simulink model "carSimulation_model"  (R2025b)
settings: Solver=VariableStepAuto  StartTime=0.0  StopTime=1000  RelTol=1e-3
settings Model: Creator=Eddy  LastModifiedBy=Eddy

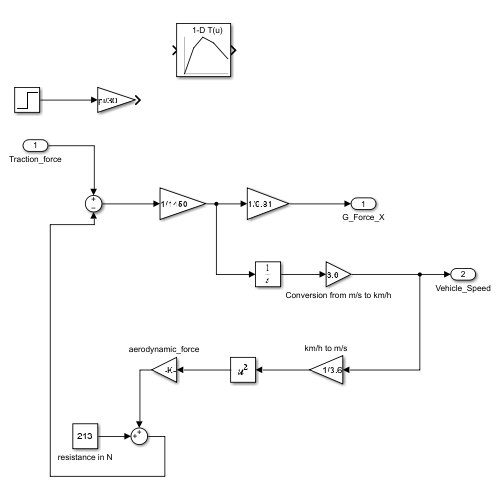
[thumbnail: Simulink's stored preview of the top-level diagram]
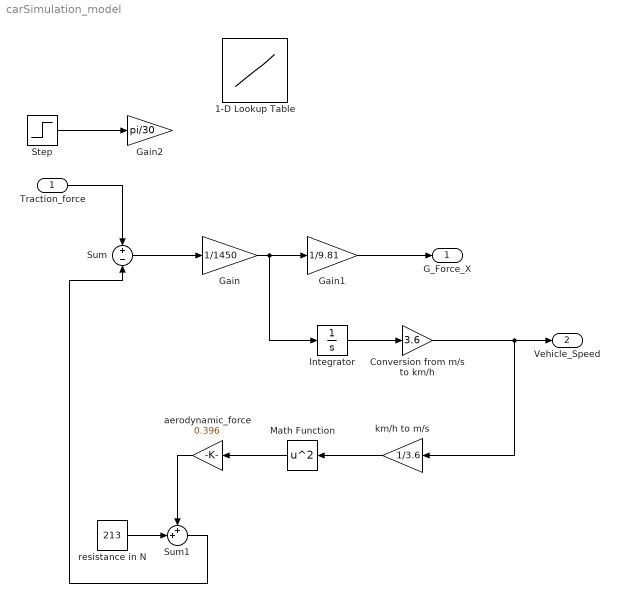
== system carSimulation_model ==
  Traction_force : Inport
  1-D Lookup Table : Lookup_n-D  NumberOfTableDimensions=1  BreakpointsForDimension1=[820, 1500, 2200, 3000, 4000]  Table="[80,  250,  320,  280,  180]"  InternalRulePriority=Speed  RndMeth=Simplest
  Conversion from m/s to km/h : Gain  Gain=3.6
  Gain : Gain  Gain=1/1450
  Gain1 : Gain  Gain=1/9.81
  Gain2 : Gain  Gain=pi/30
  Integrator : Integrator
  Math Function : Math  Operator=square
  Step : Step  SampleTime=0
  Sum : Sum  Inputs=+|-
  Sum1 : Sum  Inputs=++|
  aerodynamic_force : Gain  Gain=0.396
  km/h to m/s : Gain  Gain=1/3.6
  resistance in N : Constant  Value=213
  G_Force_X : Outport
  Vehicle_Speed : Outport  Port=2
  wires:
  Sum/1 -> Gain/1
  Gain/1 -> Integrator/1, Gain1/1
  Gain1/1 -> G_Force_X/1
  Integrator/1 -> Conversion from m/s to km/h/1
  Conversion from m/s to km/h/1 -> km/h to m/s/1, Vehicle_Speed/1
  Traction_force/1 -> Sum/1
  km/h to m/s/1 -> Math Function/1
  Math Function/1 -> aerodynamic_force/1
  resistance in N/1 -> Sum1/2
  aerodynamic_force/1 -> Sum1/1
  Sum1/1 -> Sum/2
  Step/1 -> Gain2/1
